simulink model "calibrateIMU"  (Simulink 8.6)
settings: Solver=FixedStepDiscrete  StartTime=0.0  StopTime=inf  FixedStep=0.01  RelTol=1e-3
InitFcn:
  | ROBOT_DOF=23;
libraries: WBToolboxLibrary x4
settings Model: Creator=DanielePucci  LastModifiedBy=DanielePucci
settings DataIOCC: SaveFormat=Dataset  SignalLoggingSaveFormat=Dataset
settings OptimizationCC: ExpressionDepthLimit=128
settings DebuggingCC: UnderspecifiedInitializationDetection=Simplified  MergeDetectMultiDrivingBlocksExec=error  SolverPrmCheckMsg=none  FcnCallInpInsideContextMsg=EnableAllAsError  StateNameClashWarn=none
settings HardwareCC: ProdBitPerPointer=64  ProdLargestAtomicFloat=Float  ProdIntDivRoundTo=Zero  ProdEndianess=LittleEndian  ProdWordSize=64  ProdHWDeviceType=Intel->x86-64 (Windows64)
settings GRTTargetCC: GeneratePreprocessorConditionals=Use local settings  CombineOutputUpdateFcns=on  GRTInterface=off
settings ConfigComp: CovModelRefEnable=off

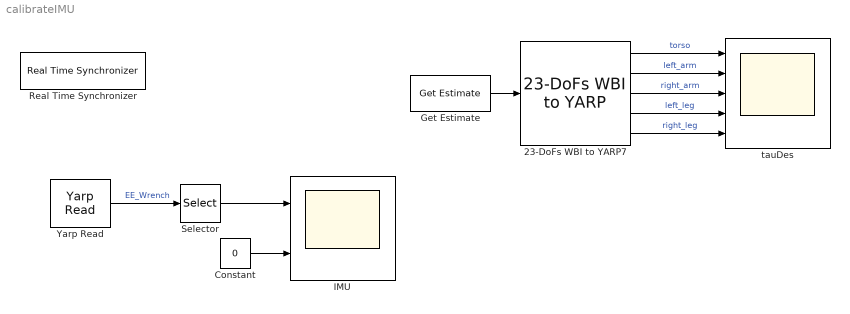
== system calibrateIMU ==
  23-DoFs WBI to YARP7 : WBToolboxLibrary/Utilities/23-DoFs WBI to YARP
  Constant : Constant  Value=0
  Get Estimate : WBToolboxLibrary/wholeBodyStates/Get Estimate  estimateType=Joints Torque  robotName=WBT_robotName  localName=WBT_modelName  wbiFile=WBT_wbiFilename  wbiList=WBT_wbiList
  IMU : Scope  NumInputPorts=2
  Real Time Synchronizer : WBToolboxLibrary/Utilities/Real Time Synchronizer  period=0.01
  Selector : Selector  InputPortWidth=12  IndexOptions=Index vector (dialog)  Indices=[4:6]  OutputSizes=1
  Yarp Read : WBToolboxLibrary/Utilities/Yarp Read  portName='/icub/inertial'  signalSize=12  blocking=off  timestamp=off  autoconnect=on  errorOnConnection=off
  tauDes : Scope  NumInputPorts=5
  wires:
  Yarp Read/1 -> Selector/1  "EE_Wrench"
  Selector/1 -> IMU/1
  Constant/1 -> IMU/2
  23-DoFs WBI to YARP7/5 -> tauDes/5  "right_leg"
  23-DoFs WBI to YARP7/1 -> tauDes/1  "torso"
  23-DoFs WBI to YARP7/2 -> tauDes/2  "left_arm"
  23-DoFs WBI to YARP7/4 -> tauDes/4  "left_leg"
  23-DoFs WBI to YARP7/3 -> tauDes/3  "right_arm"
  Get Estimate/1 -> 23-DoFs WBI to YARP7/1
